simulink model "simulink Pendulum"  (R2019a)
settings: Solver=VariableStepAuto  StartTime=0.0  StopTime=stoptime  MaxStep=maxsize  RelTol=1e-3
values from neighbouring files (symbols this model uses):
  g = 9.8    [script_file Pendulum.m]
  L = valueoflength(i)    [script_file Pendulum.m]
settings Model: Creator=MahMoud  LastModifiedBy=MahMoud

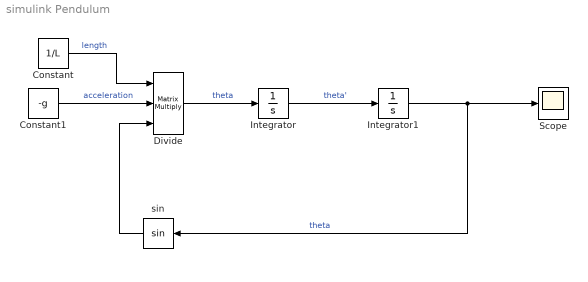
== system simulink Pendulum ==
  Constant : Constant  Value=1/L
  Constant1 : Constant  Value=-g
  Divide : Product  Inputs=***  Multiplication=Matrix(*)
  Integrator : Integrator  InitialCondition=1
  Integrator1 : Integrator  InitialCondition=1
  Scope : Scope
  sin : Trigonometry
  wires:
  Integrator/1 -> Integrator1/1  "theta'"
  sin/1 -> Divide/3
  Constant1/1 -> Divide/2  "acceleration"
  Constant/1 -> Divide/1  "length"
  Divide/1 -> Integrator/1  "theta"
  Integrator1/1 -> sin/1, Scope/1  "theta"
